simulink library "sm_excv_underc_lib"  (R2023b)
settings: Solver=VariableStepAuto  StartTime=0.0  StopTime=10.0  RelTol=1e-3
undefined symbols (not defined in the file): Excv, L1, L2, L3, L4, L5, L6, L7, L8, L9, P1, P2, P3, P4, P5, P6, P7, P8, P9, shoe_w, X, Y, Z
libraries: sm_tracked_vehicle_lib x70, sm_lib x54, nesl_utility x32, sm_excv_scene_lib x9, fl_lib x8, sm_excv_frame_lib x4
(part 3 of 5)

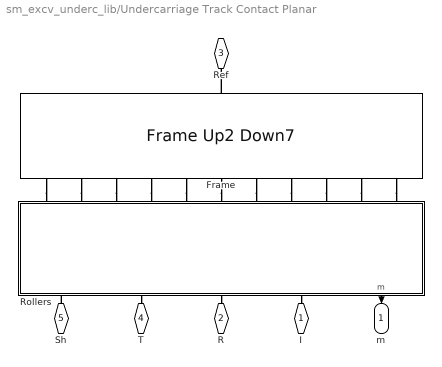
== system sm_excv_underc_lib/Undercarriage Track Contact Planar ==
  Frame : sm_excv_frame_lib/Frame Up2 Down7  roller_upper_x=roller_upper_x  roller_lower_x=roller_lower_x  idler_x=idler_x  roller_upper_y=roller_upper_y  sprk_pitch_rad=sprk_pitch_rad  roller_lower_rad=roller_lower_rad  plate_h=plate_h  idler_rad=idler_rad  idler_lower_roller_offset_y=idler_lower_roller_offset_y
  Rollers : Subsystem  mask(Rollers for Integration with Track Model){sprk_xc=sprk_xc, sprk_len=sprk_len, sprk_rho=sprk_rho, sprk_clr=sprk_clr, sprk_opc=sprk_opc, sprk_contact_geo_ptcld=sprk_contact_geo_ptcld, sprk_contact_geo_rad=sprk_contact_geo_rad, sprk_contact_geo_clr=sprk_contact_geo_clr, sprk_contact_geo_opc=sprk_contact_geo_opc, idler_rad=idler_rad, idler_len=idler_len, idler_rho=idler_rho, idler_clr=idler_clr, idler_opc=idler_opc, idler_contgeo_clr=idler_contgeo_clr, idler_contgeo_opc=idler_contgeo_opc, roller_upper_len=roller_upper_len, roller_upper_rad=roller_upper_rad, roller_upper_rho=roller_upper_rho, roller_upper_clr=roller_upper_clr, roller_upper_opc=roller_upper_opc, roller_upper_contgeo_clr=roller_upper_contgeo_clr, roller_upper_contgeo_opc=roller_upper_contgeo_opc, roller_lower_len=roller_lower_len, roller_lower_rad=roller_lower_rad, roller_lower_rho=roller_lower_rho, roller_lower_clr=roller_lower_clr, roller_lower_opc=roller_lower_opc, roller_lower_contgeo_clr=roller_lower_contgeo_clr, roller_lower_contgeo_opc=roller_lower_contgeo_opc, tensioner_cyl_rad=tensioner_cyl_rad, tensioner_cyl_len=tensioner_cyl_len, tensioner_cyl_rho=tensioner_cyl_rho, tensioner_cyl_clr=tensioner_cyl_clr, tensioner_cyl_opc=tensioner_cyl_opc, tensioner_pist_rad=tensioner_pist_rad, tensioner_pist_len=tensioner_pist_len, tensioner_pist_rho=tensioner_pist_rho, tensioner_pist_clr=tensioner_pist_clr, tensioner_pist_opc=tensioner_pist_opc, tensioner_br_length=tensioner_br_length, tensioner_br_width=tensioner_br_width, tensioner_br_height=tensioner_br_height, tensioner_br_thk=tensioner_br_thk, tensioner_br_rho=tensioner_br_rho, tensioner_br_clr=tensioner_br_clr, tensioner_br_opc=tensioner_br_opc, tensioner_eqpos=tensioner_eqpos, tensioner_x0=tensioner_x0, tensioner_b=tensioner_b, tensioner_k=tensioner_k, popup_sense_roller=Actuator Torque}
      mask prompts: sprk_xc "Extrusion Data [x y] (m)"; sprk_len "Length (m)"; sprk_rho "Density (kg/m^3)"; sprk_clr "Color [R G B] (0-1)"; sprk_opc "Opacity (0-1)"; sprk_contact_geo_ptcld "Point Cloud Data [x y z] (m)"; sprk_contact_geo_rad "Radius (m)"; sprk_contact_geo_clr "Color [R G B] (0-1)"; sprk_contact_geo_opc "Opacity (0-1)"; idler_rad "Radius (m)"; idler_len "Length(m)"; idler_rho "Density (kg/m^3)"; idler_clr "Color [R G B] (0-1)"; idler_opc "Opacity (0-1)"; idler_contgeo_clr "Color [R G B] (0-1)"; idler_contgeo_opc "Opacity (0-1)"; roller_upper_len "Length (m)"; roller_upper_rad "Radius (m)"; roller_upper_rho "Density (kg/m^3)"; roller_upper_clr "Color [R G B] (0-1)"; roller_upper_opc "Opacity (0-1)"; roller_upper_contgeo_clr "Color [R G B] (0-1)"; roller_upper_contgeo_opc "Opacity (0-1)"; roller_lower_len "Length (m)"; roller_lower_rad "Radius (m)"; roller_lower_rho "Density (kg/m^3)"; roller_lower_clr "Color [R G B] (0-1)"; roller_lower_opc "Opacity (0-1)"; roller_lower_contgeo_clr "Color [R G B] (0-1)"; roller_lower_contgeo_opc "Opacity (0-1)"; tensioner_cyl_rad "Radius (m)"; tensioner_cyl_len "Length (m)"; tensioner_cyl_rho "Density (kg/m^3)"; tensioner_cyl_clr "Color [R G B] (0-1)"; tensioner_cyl_opc "Opacity (0-1)"; tensioner_pist_rad "Radius (m)"; tensioner_pist_len "Length (m)"; tensioner_pist_rho "Density (kg/m^3)"; tensioner_pist_clr "Color [R G B] (0-1)"; tensioner_pist_opc "Opacity (0.1)"; tensioner_br_length "Length (m)"; tensioner_br_width "Width (m)"; tensioner_br_height "Height (m)"; tensioner_br_thk "Thickness (m)"; tensioner_br_rho "Density (kg/m^3)"; tensioner_br_clr "Color [R G B] (0-1)"; tensioner_br_opc "Opacity (0.1)"; tensioner_eqpos "Equilibrium Position (m)"; tensioner_x0 "Assembly Position (m)"; tensioner_b "Damping Coefficient (N/(m/s))"; tensioner_k "Stiffness Coefficient (N/m)"; popup_sense_roller "Roller"
      mask help: Models sprocket, rollers, and idler with tensioner. Components have contact geometry for integration with a segmented track model. Contact forces within the track are planar to speed up simulation. The sprocket has a 1D rotational mechanical interface to the drivetrain.
      mask init: same as sm_excv_underc_lib/Undercarriage Roller Contact Sphere/Rollers
      mask TypeOptions sprk_xc: Sprocket/sprk_xc
      mask TypeOptions sprk_len: Sprocket/sprk_len
      mask TypeOptions sprk_rho: Sprocket/sprk_rho
      mask TypeOptions sprk_clr: Sprocket/sprk_clr
      mask TypeOptions sprk_opc: Sprocket/sprk_opc
      mask TypeOptions sprk_contact_geo_ptcld: Sprocket/sprk_contact_geo_ptcld
      mask TypeOptions sprk_contact_geo_rad: Sprocket/sprk_contact_geo_rad
      mask TypeOptions sprk_contact_geo_clr: Sprocket/sprk_contact_geo_clr
      mask TypeOptions sprk_contact_geo_opc: Sprocket/sprk_contact_geo_opc
      mask TypeOptions idler_rad: Idler/idler_rad
      mask TypeOptions idler_len: Idler/idler_len
      mask TypeOptions idler_rho: Idler/idler_rho
      mask TypeOptions idler_clr: Idler/idler_clr
      mask TypeOptions idler_opc: Idler/idler_opc
      mask TypeOptions idler_contgeo_clr: Idler/idler_contgeo_clr
      mask TypeOptions idler_contgeo_opc: Idler/idler_contgeo_opc
      mask TypeOptions roller_upper_len:
      | Roller
      | Upper 1/roller_upper_len | Roller
      | Upper 2/roller_upper_len
      mask TypeOptions roller_upper_rad:
      | Roller
      | Upper 1/roller_upper_rad | Roller
      | Upper 2/roller_upper_rad
      mask TypeOptions roller_upper_rho:
      | Roller
      | Upper 1/roller_upper_rho | Roller
      | Upper 2/roller_upper_rho
      mask TypeOptions roller_upper_clr:
      | Roller
      | Upper 1/roller_upper_clr | Roller
      | Upper 2/roller_upper_clr
      mask TypeOptions roller_upper_opc:
      | Roller
      | Upper 1/roller_upper_opc | Roller
      | Upper 2/roller_upper_opc
      mask TypeOptions roller_upper_contgeo_clr:
      | Roller
      | Upper 1/roller_upper_contgeo_clr | Roller
      | Upper 2/roller_upper_contgeo_clr
      mask TypeOptions roller_upper_contgeo_opc:
      | Roller
      | Upper 1/roller_upper_contgeo_opc | Roller
      | Upper 2/roller_upper_contgeo_opc
      mask TypeOptions roller_lower_len:
      | Roller
      | Lower 1/roller_lower_len | Roller
      | Lower 2/roller_lower_len | Roller
      | Lower 3/roller_lower_len | Roller
      | Lower 4/roller_lower_len | Roller
      | Lower 5/roller_lower_len | Roller
      | Lower 6/roller_lower_len | Roller
      | Lower 7/roller_lower_len
      mask TypeOptions roller_lower_rad:
      | Roller
      | Lower 1/roller_lower_rad | Roller
      | Lower 2/roller_lower_rad | Roller
      | Lower 3/roller_lower_rad | Roller
      | Lower 4/roller_lower_rad | Roller
      | Lower 5/roller_lower_rad | Roller
      | Lower 6/roller_lower_rad | Roller
      | Lower 7/roller_lower_rad
      mask TypeOptions roller_lower_rho:
      | Roller
      | Lower 1/roller_lower_rho | Roller
      | Lower 2/roller_lower_rho | Roller
      | Lower 3/roller_lower_rho | Roller
      | Lower 4/roller_lower_rho | Roller
      | Lower 5/roller_lower_rho | Roller
      | Lower 6/roller_lower_rho | Roller
      | Lower 7/roller_lower_rho
      mask TypeOptions roller_lower_clr:
      | Roller
      | Lower 1/roller_lower_clr | Roller
      | Lower 2/roller_lower_clr | Roller
      | Lower 3/roller_lower_clr | Roller
      | Lower 4/roller_lower_clr | Roller
      | Lower 5/roller_lower_clr | Roller
      | Lower 6/roller_lower_clr | Roller
      | Lower 7/roller_lower_clr
      mask TypeOptions roller_lower_opc:
      | Roller
      | Lower 1/roller_lower_opc | Roller
      | Lower 2/roller_lower_opc | Roller
      | Lower 3/roller_lower_opc | Roller
      | Lower 4/roller_lower_opc | Roller
      | Lower 5/roller_lower_opc | Roller
      | Lower 6/roller_lower_opc | Roller
      | Lower 7/roller_lower_opc
      mask TypeOptions roller_lower_contgeo_clr:
      | Roller
      | Lower 1/roller_lower_contgeo_clr | Roller
      | Lower 2/roller_lower_contgeo_clr | Roller
      | Lower 3/roller_lower_contgeo_clr | Roller
      | Lower 4/roller_lower_contgeo_clr | Roller
      | Lower 5/roller_lower_contgeo_clr | Roller
      | Lower 6/roller_lower_contgeo_clr | Roller
      | Lower 7/roller_lower_contgeo_clr
      mask TypeOptions roller_lower_contgeo_opc:
      | Roller
      | Lower 1/roller_lower_contgeo_opc | Roller
      | Lower 2/roller_lower_contgeo_opc | Roller
      | Lower 3/roller_lower_contgeo_opc | Roller
      | Lower 4/roller_lower_contgeo_opc | Roller
      | Lower 5/roller_lower_contgeo_opc | Roller
      | Lower 6/roller_lower_contgeo_opc | Roller
      | Lower 7/roller_lower_contgeo_opc
      mask TypeOptions tensioner_cyl_rad:
      | Tensioner
      | Cylinder/cyl_rad
      mask TypeOptions tensioner_cyl_len:
      | Tensioner
      | Cylinder/cyl_len
      mask TypeOptions tensioner_cyl_rho:
      | Tensioner
      | Cylinder/cyl_rho
      mask TypeOptions tensioner_cyl_clr:
      | Tensioner
      | Cylinder/cyl_clr
      mask TypeOptions tensioner_cyl_opc:
      | Tensioner
      | Cylinder/cyl_opc
      mask TypeOptions tensioner_pist_rad:
      | Tensioner
      | Piston/pist_rad
      mask TypeOptions tensioner_pist_len:
      | Tensioner
      | Piston/pist_len
      mask TypeOptions tensioner_pist_rho:
      | Tensioner
      | Piston/pist_rho
      mask TypeOptions tensioner_pist_clr:
      | Tensioner
      | Piston/pist_clr
      mask TypeOptions tensioner_pist_opc:
      | Tensioner
      | Piston/pist_opc
      mask TypeOptions tensioner_br_length:
      | Tensioner
      | Piston/br_length
      mask TypeOptions tensioner_br_width:
      | Tensioner
      | Piston/br_width
      mask TypeOptions tensioner_br_height:
      | Tensioner
      | Piston/br_height
      mask TypeOptions tensioner_br_thk:
      | Tensioner
      | Piston/br_thk
      mask TypeOptions tensioner_br_rho:
      | Tensioner
      | Piston/br_rho
      mask TypeOptions tensioner_br_clr:
      | Tensioner
      | Piston/br_clr
      mask TypeOptions tensioner_br_opc:
      | Tensioner
      | Piston/br_opc
      mask TypeOptions tensioner_eqpos:
      | Prismatic
      | Tensioner/EquilibriumPosition
      mask TypeOptions tensioner_x0:
      | Prismatic
      | Tensioner/PositionTargetValue
      mask TypeOptions tensioner_b:
      | Prismatic
      | Tensioner/DampingCoefficient
      mask TypeOptions tensioner_k:
      | Prismatic
      | Tensioner/SpringStiffness
      mask TypeOptions popup_sense_roller: Constraint Force | Actuator Torque
      mask DialogControl cont_sprk Prompt: Sprocket
      mask DialogControl cont_sprk_solid Prompt: Solid
      mask DialogControl cont_sprk_contact_geo Prompt: Contact Geometry
      mask DialogControl cont_idler Prompt: Idler
      mask DialogControl cont_idler_solid Prompt: Solid
      mask DialogControl cont_idler_contact_geo Prompt: Contact Geometry
      mask DialogControl cont_rollers Prompt: Rollers
      mask DialogControl cont_roller_upper Prompt: Upper
      mask DialogControl cont_roller_upper_contact_geo Prompt: Contact Geometry
      mask DialogControl cont_lower Prompt: Lower
      mask DialogControl cont_lower_contact_geo Prompt: Contact Geometry
      mask DialogControl cont_tensioner Prompt: Tensioner
      mask DialogControl cont_tensioner_cyl Prompt: Cylinder
      mask DialogControl cont_tensioner_pist Prompt: Piston
      mask DialogControl cont_tensioner_brkt Prompt: Bracket
      mask DialogControl cont_tensioner_assy Prompt: Assembly
      mask DialogControl cont_sensing Prompt: Sensing
      mask Display:
      | image('sm_excv_track_rollers_IMAGE.png');
      | disp('Pla')
  I : PMIOPort  Side=Right
  R : PMIOPort  Port=2  Side=Right
  Ref : PMIOPort  Port=3  Side=Right
  T : PMIOPort  Port=4  Side=Right
  Sh : PMIOPort  Port=5  Side=Right
  m : Outport
  wires:
  Rollers/1(m) -> m/1
  connections:
  Sh/RConn1 -- Rollers/RConn4
  Frame/RConn2 -- Rollers/LConn2
  Frame/RConn3 -- Rollers/LConn3
  Frame/RConn11 -- Rollers/LConn11
  Frame/RConn1 -- Rollers/LConn1
  Frame/RConn6 -- Rollers/LConn6
  Frame/RConn9 -- Rollers/LConn9
  Frame/RConn10 -- Rollers/LConn10
  Frame/RConn8 -- Rollers/LConn8
  Frame/RConn4 -- Rollers/LConn4
  Frame/RConn5 -- Rollers/LConn5
  Frame/RConn7 -- Rollers/LConn7
  Rollers/RConn3 -- T/RConn1
  Rollers/RConn1 -- I/RConn1
  Frame/LConn1 -- Ref/RConn1
  Rollers/RConn2 -- R/RConn1

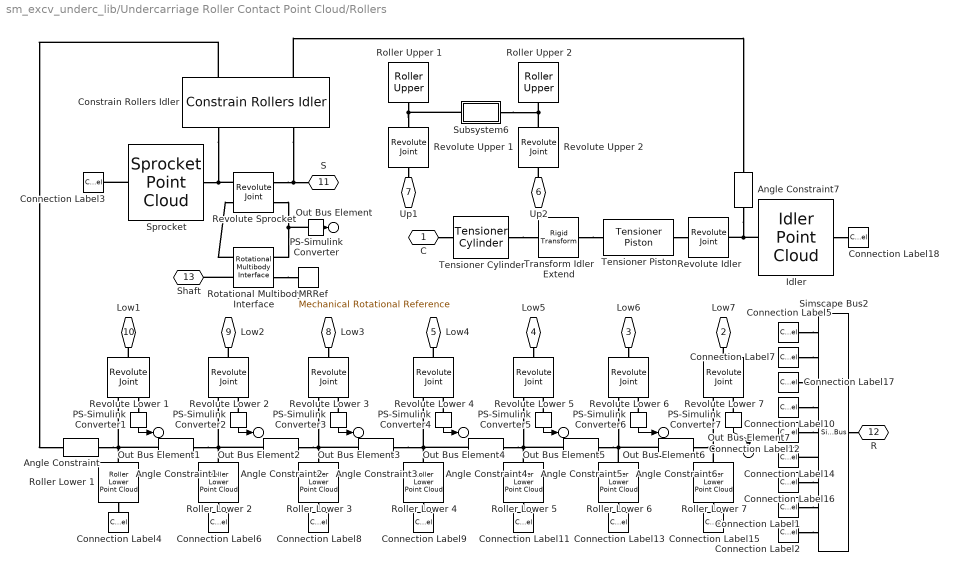
== system sm_excv_underc_lib/Undercarriage Roller Contact Point Cloud/Rollers ==
  Angle Constraint{,1..7} (8 alike) : sm_tracked_vehicle_lib/Angle Constraint  SystemSampleTime=-1  VariantActivationTime=update diagram  AllowFlexibleInterface=on  Latency=0  AutoFrameSizeCalculation=off
  Connection Label1 : ConnectionLabel  Label=Spr
  Connection Label10 : ConnectionLabel  Label=L4
  Connection Label11 : ConnectionLabel  Label=L5
  Connection Label12 : ConnectionLabel  Label=L5
  Connection Label13 : ConnectionLabel  Label=L6
  Connection Label14 : ConnectionLabel  Label=L6
  Connection Label15 : ConnectionLabel  Label=L7
  Connection Label16 : ConnectionLabel  Label=L7
  Connection Label17 : ConnectionLabel  Label=L3
  Connection Label18 : ConnectionLabel  Label=Idl
  Connection Label2 : ConnectionLabel  Label=Idl
  Connection Label3 : ConnectionLabel  Label=Spr
  Connection Label4 : ConnectionLabel  Label=L1
  Connection Label5 : ConnectionLabel  Label=L1
  Connection Label6 : ConnectionLabel  Label=L2
  Connection Label7 : ConnectionLabel  Label=L2
  Connection Label8 : ConnectionLabel  Label=L3
  Connection Label9 : ConnectionLabel  Label=L4
  Constrain Rollers Idler : sm_tracked_vehicle_lib/Constrain Rollers Idler  sprk_rolling_rad=sprk_rolling_rad  roller_lower_rolling_rad=roller_lower_rolling_rad  idler_rolling_rad=idler_rolling_rad
  Idler : sm_tracked_vehicle_lib/Idler Point Cloud  idler_rad=idler_rad  idler_len=idler_len  idler_rho=idler_rho  idler_clr=idler_clr  idler_opc=idler_opc  idler_contact_geo_ptcld=idler_contact_geo_ptcld  idler_contact_geo_rad=idler_contact_geo_rad  idler_contact_geo_clr=idler_contact_geo_clr  idler_contact_geo_opc=idler_contact_geo_opc  cyl_rad=idler_rolling_rad  cyl_len=cyl_len  cyl_clr=idler_cyl_clr  cyl_opc=idler_cyl_opc  accMn=accMn  accMx=accMx  acc_clr=acc_clr  acc_opc=acc_opc  lext=lext
  MRRef : fl_lib/Mechanical/Rotational Elements/Mechanical Rotational Reference
  PS-Simulink Converter{,1..7} (8 alike) : nesl_utility/PS-Simulink Converter  PhysicalDomain=network_engine_domain  SubClassName=ps_output  LeftPortType=input  RightPortType=output  PseudoPeriodic=off  Frequencies=[]  VectorFormat=inherit  Unit=inherit  AffineConversion=off
  Revolute Idler : sm_lib/Joints/Revolute Joint  JointMode=Normal  SenseConstraintForce=off  SenseConstraintForceX=off  SenseConstraintForceY=off  SenseConstraintForceZ=off  SenseConstraintTorque=off  SenseConstraintTorqueX=off  SenseConstraintTorqueY=off  SenseConstraintTorqueZ=off  SenseTotalForce=off  SenseTotalForceX=off  SenseTotalForceY=off  SenseTotalForceZ=off  SenseTotalTorque=off  SenseTotalTorqueX=off  SenseTotalTorqueY=off  SenseTotalTorqueZ=off  CompositeWrenchDir=FollowerOnBase  CompositeWrenchFrame=BaseFrame  EquilibriumPosition=0  EquilibriumPositionUnits=rad  SpringStiffness=0  SpringStiffnessUnits=N*m/rad  DampingCoefficient=0  DampingCoefficientUnits=N*m/(rad/s)  TorqueActuationMode=NoTorque  MotionActuationMode=ComputedMotion  SensePosition=off  SenseVelocity=off  SenseAcceleration=off  SenseTorqueForce=off  SenseLowerLimitTorqueForce=off  SenseUpperLimitTorqueForce=off  LowerLimitSpecify=off  LowerLimitBound=-90  LowerLimitBoundUnits=deg  LowerLimitStiffness=1e4  LowerLimitStiffnessUnits=N*m/deg  LowerLimitDamping=10  LowerLimitDampingUnits=N*m/(deg/s)  LowerLimitTransitionRegionWidth=0.1  LowerLimitTransitionRegionWidthUnits=deg  UpperLimitSpecify=off  UpperLimitBound=90  UpperLimitBoundUnits=deg  UpperLimitStiffness=1e4  UpperLimitStiffnessUnits=N*m/deg  UpperLimitDamping=10  UpperLimitDampingUnits=N*m/(deg/s)  UpperLimitTransitionRegionWidth=0.1  UpperLimitTransitionRegionWidthUnits=deg  PositionTargetSpecify=off  PositionTargetPriority=Low  PositionTargetValue=0  PositionTargetValueUnits=deg  VelocityTargetSpecify=off  VelocityTargetPriority=High  VelocityTargetValue=0  VelocityTargetValueUnits=deg/s
  Revolute Lower {1..7} (7 alike) : sm_lib/Joints/Revolute Joint  JointMode=Normal  SenseConstraintForce=off  SenseConstraintForceX=off  SenseConstraintForceY=off  SenseConstraintForceZ=off  SenseConstraintTorque=off  SenseConstraintTorqueX=off  SenseConstraintTorqueY=off  SenseConstraintTorqueZ=off  SenseTotalForce=off  SenseTotalForceX=off  SenseTotalForceY=off  SenseTotalForceZ=off  SenseTotalTorque=off  SenseTotalTorqueX=off  SenseTotalTorqueY=off  SenseTotalTorqueZ=off  CompositeWrenchDir=FollowerOnBase  CompositeWrenchFrame=BaseFrame  EquilibriumPosition=0  EquilibriumPositionUnits=rad  SpringStiffness=0  SpringStiffnessUnits=N*m/rad  DampingCoefficient=0  DampingCoefficientUnits=N*m/(rad/s)  TorqueActuationMode=NoTorque  MotionActuationMode=ComputedMotion  SensePosition=off  SenseVelocity=off  SenseAcceleration=off  SenseTorqueForce=on  SenseLowerLimitTorqueForce=off  SenseUpperLimitTorqueForce=off  LowerLimitSpecify=off  LowerLimitBound=-90  LowerLimitBoundUnits=deg  LowerLimitStiffness=1e4  LowerLimitStiffnessUnits=N*m/deg  LowerLimitDamping=10  LowerLimitDampingUnits=N*m/(deg/s)  LowerLimitTransitionRegionWidth=0.1  LowerLimitTransitionRegionWidthUnits=deg  UpperLimitSpecify=off  UpperLimitBound=90  UpperLimitBoundUnits=deg  UpperLimitStiffness=1e4  UpperLimitStiffnessUnits=N*m/deg  UpperLimitDamping=10  UpperLimitDampingUnits=N*m/(deg/s)  UpperLimitTransitionRegionWidth=0.1  UpperLimitTransitionRegionWidthUnits=deg  PositionTargetSpecify=off  PositionTargetPriority=Low  PositionTargetValue=0  PositionTargetValueUnits=deg  VelocityTargetSpecify=off  VelocityTargetPriority=High  VelocityTargetValue=0  VelocityTargetValueUnits=deg/s
  Revolute Sprocket : sm_lib/Joints/Revolute Joint  JointMode=Normal  SenseConstraintForce=off  SenseConstraintForceX=off  SenseConstraintForceY=off  SenseConstraintForceZ=off  SenseConstraintTorque=off  SenseConstraintTorqueX=off  SenseConstraintTorqueY=off  SenseConstraintTorqueZ=off  SenseTotalForce=off  SenseTotalForceX=off  SenseTotalForceY=off  SenseTotalForceZ=off  SenseTotalTorque=off  SenseTotalTorqueX=off  SenseTotalTorqueY=off  SenseTotalTorqueZ=off  CompositeWrenchDir=FollowerOnBase  CompositeWrenchFrame=BaseFrame  EquilibriumPosition=0  EquilibriumPositionUnits=rad  SpringStiffness=0  SpringStiffnessUnits=N*m/rad  DampingCoefficient=0  DampingCoefficientUnits=N*m/(rad/s)  TorqueActuationMode=InputTorque  MotionActuationMode=ComputedMotion  SensePosition=off  SenseVelocity=on  SenseAcceleration=off  SenseTorqueForce=off  SenseLowerLimitTorqueForce=off  SenseUpperLimitTorqueForce=off  LowerLimitSpecify=off  LowerLimitBound=-90  LowerLimitBoundUnits=deg  LowerLimitStiffness=1e4  LowerLimitStiffnessUnits=N*m/deg  LowerLimitDamping=10  LowerLimitDampingUnits=N*m/(deg/s)  LowerLimitTransitionRegionWidth=0.1  LowerLimitTransitionRegionWidthUnits=deg  UpperLimitSpecify=off  UpperLimitBound=90  UpperLimitBoundUnits=deg  UpperLimitStiffness=1e4  UpperLimitStiffnessUnits=N*m/deg  UpperLimitDamping=10  UpperLimitDampingUnits=N*m/(deg/s)  UpperLimitTransitionRegionWidth=0.1  UpperLimitTransitionRegionWidthUnits=deg  PositionTargetSpecify=off  PositionTargetPriority=Low  PositionTargetValue=0  PositionTargetValueUnits=deg  VelocityTargetSpecify=off  VelocityTargetPriority=High  VelocityTargetValue=0  VelocityTargetValueUnits=deg/s
  Revolute Upper 1 : sm_lib/Joints/Revolute Joint  JointMode=Normal  SenseConstraintForce=off  SenseConstraintForceX=off  SenseConstraintForceY=off  SenseConstraintForceZ=off  SenseConstraintTorque=off  SenseConstraintTorqueX=off  SenseConstraintTorqueY=off  SenseConstraintTorqueZ=off  SenseTotalForce=off  SenseTotalForceX=off  SenseTotalForceY=off  SenseTotalForceZ=off  SenseTotalTorque=off  SenseTotalTorqueX=off  SenseTotalTorqueY=off  SenseTotalTorqueZ=off  CompositeWrenchDir=FollowerOnBase  CompositeWrenchFrame=BaseFrame  EquilibriumPosition=0  EquilibriumPositionUnits=rad  SpringStiffness=0  SpringStiffnessUnits=N*m/rad  DampingCoefficient=0  DampingCoefficientUnits=N*m/(rad/s)  TorqueActuationMode=NoTorque  MotionActuationMode=ComputedMotion  SensePosition=off  SenseVelocity=off  SenseAcceleration=off  SenseTorqueForce=off  SenseLowerLimitTorqueForce=off  SenseUpperLimitTorqueForce=off  LowerLimitSpecify=off  LowerLimitBound=-90  LowerLimitBoundUnits=deg  LowerLimitStiffness=1e4  LowerLimitStiffnessUnits=N*m/deg  LowerLimitDamping=10  LowerLimitDampingUnits=N*m/(deg/s)  LowerLimitTransitionRegionWidth=0.1  LowerLimitTransitionRegionWidthUnits=deg  UpperLimitSpecify=off  UpperLimitBound=90  UpperLimitBoundUnits=deg  UpperLimitStiffness=1e4  UpperLimitStiffnessUnits=N*m/deg  UpperLimitDamping=10  UpperLimitDampingUnits=N*m/(deg/s)  UpperLimitTransitionRegionWidth=0.1  UpperLimitTransitionRegionWidthUnits=deg  PositionTargetSpecify=off  PositionTargetPriority=Low  PositionTargetValue=0  PositionTargetValueUnits=deg  VelocityTargetSpecify=off  VelocityTargetPriority=High  VelocityTargetValue=0  VelocityTargetValueUnits=deg/s
  Revolute Upper 2 : sm_lib/Joints/Revolute Joint  JointMode=Normal  SenseConstraintForce=off  SenseConstraintForceX=off  SenseConstraintForceY=off  SenseConstraintForceZ=off  SenseConstraintTorque=off  SenseConstraintTorqueX=off  SenseConstraintTorqueY=off  SenseConstraintTorqueZ=off  SenseTotalForce=off  SenseTotalForceX=off  SenseTotalForceY=off  SenseTotalForceZ=off  SenseTotalTorque=off  SenseTotalTorqueX=off  SenseTotalTorqueY=off  SenseTotalTorqueZ=off  CompositeWrenchDir=FollowerOnBase  CompositeWrenchFrame=BaseFrame  EquilibriumPosition=0  EquilibriumPositionUnits=rad  SpringStiffness=0  SpringStiffnessUnits=N*m/rad  DampingCoefficient=0  DampingCoefficientUnits=N*m/(rad/s)  TorqueActuationMode=NoTorque  MotionActuationMode=ComputedMotion  SensePosition=off  SenseVelocity=off  SenseAcceleration=off  SenseTorqueForce=off  SenseLowerLimitTorqueForce=off  SenseUpperLimitTorqueForce=off  LowerLimitSpecify=off  LowerLimitBound=-90  LowerLimitBoundUnits=deg  LowerLimitStiffness=1e4  LowerLimitStiffnessUnits=N*m/deg  LowerLimitDamping=10  LowerLimitDampingUnits=N*m/(deg/s)  LowerLimitTransitionRegionWidth=0.1  LowerLimitTransitionRegionWidthUnits=deg  UpperLimitSpecify=off  UpperLimitBound=90  UpperLimitBoundUnits=deg  UpperLimitStiffness=1e4  UpperLimitStiffnessUnits=N*m/deg  UpperLimitDamping=10  UpperLimitDampingUnits=N*m/(deg/s)  UpperLimitTransitionRegionWidth=0.1  UpperLimitTransitionRegionWidthUnits=deg  PositionTargetSpecify=off  PositionTargetPriority=Low  PositionTargetValue=0  PositionTargetValueUnits=deg  VelocityTargetSpecify=off  VelocityTargetPriority=High  VelocityTargetValue=0  VelocityTargetValueUnits=deg/s
  Roller Lower {1..7} (7 alike) : sm_tracked_vehicle_lib/Roller Lower Point Cloud  roller_lower_rad=roller_lower_rad  roller_lower_len=roller_lower_len  roller_lower_rho=roller_lower_rho  roller_lower_clr=roller_lower_clr  roller_lower_opc=roller_lower_opc  roller_lower_contgeo_ptcld=roller_lower_contgeo_ptcld  roller_lower_contgeo_rad=roller_lower_contgeo_rad  roller_lower_contgeo_clr=roller_lower_contgeo_clr  roller_lower_contgeo_opc=roller_lower_contgeo_opc  cyl_rad=roller_lower_rolling_rad  cyl_len=cyl_len  cyl_clr=roller_cyl_clr  cyl_opc=roller_cyl_opc  accMn=accMn  accMx=accMx  acc_clr=acc_clr  acc_opc=acc_opc  lext=lext
      settings: LibrarySourceBlock=sm_chain_drive_lib/Pulley_Bot
  Roller Upper 1 : sm_tracked_vehicle_lib/Roller Upper  roller_upper_rad=roller_upper_rad  roller_upper_len=roller_upper_len  roller_upper_rho=roller_upper_rho  roller_upper_clr=roller_upper_clr  roller_upper_opc=roller_upper_opc  roller_upper_contgeo_clr=roller_upper_contgeo_clr  roller_upper_contgeo_opc=roller_upper_contgeo_opc
      settings: LibrarySourceBlock=sm_chain_drive_lib/Pulley_Top
  Roller Upper 2 : sm_tracked_vehicle_lib/Roller Upper  roller_upper_rad=roller_upper_rad  roller_upper_len=roller_upper_len  roller_upper_rho=roller_upper_rho  roller_upper_clr=roller_upper_clr  roller_upper_opc=roller_upper_opc  roller_upper_contgeo_clr=roller_upper_contgeo_clr  roller_upper_contgeo_opc=roller_upper_contgeo_opc
      settings: LibrarySourceBlock=sm_chain_drive_lib/Pulley_Top
  Rotational Multibody Interface : fl_lib/Mechanical/Multibody Interfaces/Rotational Multibody Interface
  Simscape Bus2 : SimscapeBus  HierarchyStrings=P1;P2;P3;P4;P5;P6;P7;P8;P9  ConnectionType=Bus: Roller_CBO
  Sprocket : sm_tracked_vehicle_lib/Sprocket Point Cloud  sprk_xc=sprk_xc  sprk_len=sprk_len  sprk_rho=sprk_rho  sprk_clr=sprk_clr  sprk_opc=sprk_opc  sprk_contact_geo_ptcld=sprk_contact_geo_ptcld  sprk_contact_geo_rad=sprk_contact_geo_rad  sprk_contact_geo_clr=sprk_contact_geo_clr  sprk_contact_geo_opc=sprk_contact_geo_opc  cyl_rad=sprk_rolling_rad  cyl_len=cyl_len  cyl_clr=sprocket_cyl_clr  cyl_opc=sprocket_cyl_opc  accMn=accMn  accMx=accMx  acc_clr=acc_clr  acc_opc=acc_opc  lext=lext
  Subsystem6 : Subsystem
  Tensioner Cylinder : sm_tracked_vehicle_lib/Tensioner Cylinder  cyl_rad=tensioner_cyl_rad  cyl_len=tensioner_cyl_len  cyl_rho=tensioner_cyl_rho  cyl_clr=tensioner_cyl_clr  cyl_opc=tensioner_cyl_opc
      settings: LibrarySourceBlock=sm_chain_drive_lib/Idler_Housing
  Tensioner Piston : sm_tracked_vehicle_lib/Tensioner Piston  pist_rad=tensioner_pist_rad  pist_len=tensioner_pist_len  pist_rho=tensioner_pist_rho  pist_clr=tensioner_pist_clr  pist_opc=tensioner_pist_opc  br_height=tensioner_br_height  br_length=tensioner_br_length  br_width=tensioner_br_width  br_rho=tensioner_br_rho  br_thk=tensioner_br_thk  br_clr=tensioner_br_clr  br_opc=tensioner_br_opc
      settings: LibrarySourceBlock=sm_chain_drive_lib/ldler_Damper
  Transform Idler Extend : sm_lib/Frames and Transforms/Rigid Transform  TranslationMethod=StandardAxis  TranslationStandardOffset=idler_max_ext  TranslationStandardOffsetUnits=m  TranslationStandardAxis=+Z  TranslationCartesianOffset=[0 0 0]  TranslationCartesianOffsetUnits=m  TranslationROffset=0  TranslationROffsetUnits=m  TranslationZOffset=0  TranslationZOffsetUnits=m  TranslationThetaOffset=0  TranslationThetaOffsetUnits=deg  RotationMethod=None  RotationAngleUnits=deg  RotationStandardAxis=+Z  RotationAngle=0.1  RotationArbitraryAxis=[0 0 1]  FollAlignAxisA=+X  BaseAlignAxisA=+Y  FollAlignAxisB=+Y  BaseAlignAxisB=+Z  RotationSequenceAxes=FollowerAxes  RotationSequence=XYX  RotationSequenceAngles=[0 0 0]  RotationSequenceAnglesUnits=deg  RotationMatrix=[1 0 0; 0 1 0; 0 0 1]  Quaternion=[1 0 0 0]
  C : PMIOPort  Side=Left
  Low7 : PMIOPort  Port=2  Side=Left
  Low6 : PMIOPort  Port=3  Side=Left
  Low5 : PMIOPort  Port=4  Side=Left
  Low4 : PMIOPort  Port=5  Side=Left
  Up2 : PMIOPort  Port=6  Side=Left
  Up1 : PMIOPort  Port=7  Side=Left
  Low3 : PMIOPort  Port=8  Side=Left
  Low2 : PMIOPort  Port=9  Side=Left
  Low1 : PMIOPort  Port=10  Side=Left
  S : PMIOPort  Port=11  Side=Left
  R : PMIOPort  Port=12  Side=Right
  Shaft : PMIOPort  Port=13  Side=Right
  Out Bus Element : Outport  PortName=m  Element=tSprk
  Out Bus Element1 : Outport  PortName=m  Element=RL1
  Out Bus Element2 : Outport  PortName=m  Element=RL2
  Out Bus Element3 : Outport  PortName=m  Element=RL3
  Out Bus Element4 : Outport  PortName=m  Element=RL4
  Out Bus Element5 : Outport  PortName=m  Element=RL5
  Out Bus Element6 : Outport  PortName=m  Element=RL6
  Out Bus Element7 : Outport  PortName=m  Element=RL7
  wires:
  PS-Simulink Converter/1 -> Out Bus Element/1
  PS-Simulink Converter1/1 -> Out Bus Element1/1
  PS-Simulink Converter2/1 -> Out Bus Element2/1
  PS-Simulink Converter3/1 -> Out Bus Element3/1
  PS-Simulink Converter4/1 -> Out Bus Element4/1
  PS-Simulink Converter5/1 -> Out Bus Element5/1
  PS-Simulink Converter6/1 -> Out Bus Element6/1
  PS-Simulink Converter7/1 -> Out Bus Element7/1
  connections:
  Rotational Multibody Interface/LConn2 -- MRRef/LConn1
  Rotational Multibody Interface/RConn2 -- Shaft/RConn1
  Rotational Multibody Interface/RConn1 -- Revolute Sprocket/RConn2
  PS-Simulink Converter/LConn1 -- Rotational Multibody Interface/LConn1 -- Revolute Sprocket/LConn2
  Up2/RConn1 -- Revolute Upper 2/LConn1
  Roller Upper 1/LConn1 -- Subsystem6/LConn1 -- Revolute Upper 1/RConn1
  Low6/RConn1 -- Revolute Lower 6/LConn1
  Angle Constraint3/RConn1 -- Angle Constraint4/LConn1 -- Roller Lower 4/LConn1 -- Revolute Lower 4/RConn1
  Angle Constraint/RConn1 -- Angle Constraint1/LConn1 -- Roller Lower 1/LConn1 -- Revolute Lower 1/RConn1
  Angle Constraint6/RConn1 -- Roller Lower 7/LConn1 -- Revolute Lower 7/RConn1
  Low3/RConn1 -- Revolute Lower 3/LConn1
  Angle Constraint1/RConn1 -- Angle Constraint2/LConn1 -- Roller Lower 2/LConn1 -- Revolute Lower 2/RConn1
  Low5/RConn1 -- Revolute Lower 5/LConn1
  Connection Label5/LConn1 -- Simscape Bus2/LConn1
  Connection Label12/LConn1 -- Simscape Bus2/LConn5
  Simscape Bus2/LConn6 -- Connection Label14/LConn1
  Connection Label16/LConn1 -- Simscape Bus2/LConn7
  Connection Label7/LConn1 -- Simscape Bus2/LConn2
  Connection Label17/LConn1 -- Simscape Bus2/LConn3
  Connection Label10/LConn1 -- Simscape Bus2/LConn4
  Revolute Lower 1/LConn1 -- Low1/RConn1
  Revolute Lower 7/LConn1 -- Low7/RConn1
  Roller Lower 3/LConn1 -- Angle Constraint3/LConn1 -- Revolute Lower 3/RConn1 -- Angle Constraint2/RConn1
  Revolute Lower 4/LConn1 -- Low4/RConn1
  Roller Lower 1/RConn1 -- Connection Label4/LConn1
  Sprocket/RConn1 -- Connection Label3/LConn1
  Tensioner Piston/RConn1 -- Revolute Idler/LConn1
  Revolute Lower 2/LConn1 -- Low2/RConn1
  Revolute Upper 2/RConn1 -- Roller Upper 2/LConn1 -- Subsystem6/RConn1
  Angle Constraint5/LConn1 -- Roller Lower 5/LConn1 -- Revolute Lower 5/RConn1 -- Angle Constraint4/RConn1
  Revolute Sprocket/RConn1 -- Constrain Rollers Idler/LConn1 -- Sprocket/LConn1
  Idler/LConn1 -- Angle Constraint7/RConn1 -- Revolute Idler/RConn1
  Simscape Bus2/RConn1 -- R/RConn1
  Roller Lower 5/RConn1 -- Connection Label11/LConn1
  Revolute Sprocket/LConn1 -- Constrain Rollers Idler/LConn2 -- S/RConn1
  Roller Lower 3/RConn1 -- Connection Label8/LConn1
  Roller Lower 6/LConn1 -- Angle Constraint6/LConn1 -- Revolute Lower 6/RConn1 -- Angle Constraint5/RConn1
  Roller Lower 7/RConn1 -- Connection Label15/LConn1
  Roller Lower 4/RConn1 -- Connection Label9/LConn1
  Revolute Upper 1/LConn1 -- Up1/RConn1
  Roller Lower 2/RConn1 -- Connection Label6/LConn1
  Roller Lower 6/RConn1 -- Connection Label13/LConn1
  Idler/RConn1 -- Connection Label18/LConn1
  Transform Idler Extend/RConn1 -- Tensioner Piston/LConn1
  C/RConn1 -- Tensioner Cylinder/LConn1
  Tensioner Cylinder/RConn1 -- Transform Idler Extend/LConn1
  Constrain Rollers Idler/RConn2 -- Angle Constraint7/LConn1
  Constrain Rollers Idler/RConn1 -- Angle Constraint/LConn1
  Connection Label1/LConn1 -- Simscape Bus2/LConn8
  Connection Label2/LConn1 -- Simscape Bus2/LConn9
  Revolute Lower 1/RConn2 -- PS-Simulink Converter1/LConn1
  PS-Simulink Converter2/LConn1 -- Revolute Lower 2/RConn2
  PS-Simulink Converter3/LConn1 -- Revolute Lower 3/RConn2
  PS-Simulink Converter4/LConn1 -- Revolute Lower 4/RConn2
  PS-Simulink Converter5/LConn1 -- Revolute Lower 5/RConn2
  PS-Simulink Converter6/LConn1 -- Revolute Lower 6/RConn2
  PS-Simulink Converter7/LConn1 -- Revolute Lower 7/RConn2
